simulink model "init_custom_mask"  (Simulink 7.3)
settings: Solver=FixedStepDiscrete  StartTime=0.0  StopTime=10.0  FixedStep=1  RelTol=1e-3
settings Model: Creator=Administrator  LastModifiedBy=hnine
settings OptimizationCC: InitFltsAndDblsToZero=on
settings DebuggingCC: SaveWithParameterizedLinksMsg=none

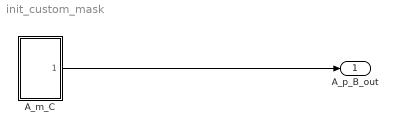
== system init_custom_mask ==
  A_m_C : Subsystem  TreatAsAtomicUnit=on  mask{A=3, B=6.7}
      mask prompts: A "Enter A:"; B "Enter B:"
      mask init:
      | C=A^2 + B^2;
  A_p_B_out : Outport  OutDataType=sfix(16)  OutScaling=2^0
  wires:
  A_m_C/1(A_m_C) -> A_p_B_out/1

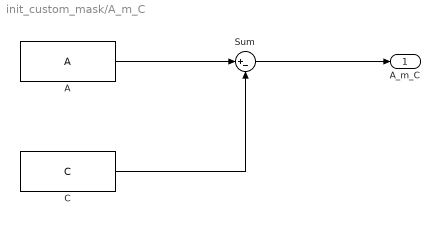
== system init_custom_mask/A_m_C ==
  A : Constant  Value=A  OutDataType=sfix(16)  OutScaling=2^0
  C : Constant  Value=C  OutDataType=sfix(16)  OutScaling=2^0
  Sum : Sum  Inputs=|+-  OutDataType=sfix(16)  OutScaling=2^0
  A_m_C : Outport  OutDataType=sfix(16)  OutScaling=2^0
  wires:
  A/1 -> Sum/1
  C/1 -> Sum/2
  Sum/1 -> A_m_C/1
